simulink model "Noncoherent_BFSK"  (R2013a)
settings: Solver=ode45  StartTime=0.0  StopTime=32/(1200)  RelTol=1e-3
libraries: commrandsrc2 x1
settings Model: Creator=Cedric  LastModifiedBy=Cedric

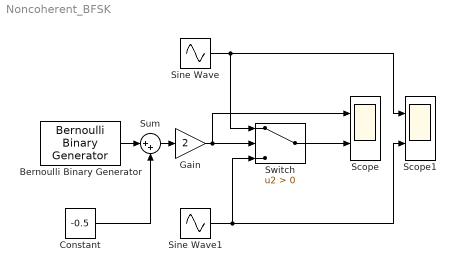
== system Noncoherent_BFSK ==
  Bernoulli Binary Generator : commrandsrc2/Bernoulli Binary Generator  P=0.5  seed=randseed  Ts=1/(1200)  frameBased=off  sampPerFrame=1  orient=off  outDataType=double
  Constant : Constant  Value=-0.5
  Gain : Gain  Gain=2
  Scope : Scope  NumInputPorts=2
      settings: YMin=-5~-5  YMax=5~5
  Scope1 : Scope  NumInputPorts=2
      settings: YMin=-5~-5  YMax=5~5
  Sine Wave : Sin  SineType=Sample based  Amplitude=5  Frequency=2*pi*1200  Samples=64  SampleTime=1/(1200*64)
  Sine Wave1 : Sin  SineType=Sample based  Amplitude=5  Frequency=2*pi*2200  Samples=64  SampleTime=1/(2200*64)
  Sum : Sum  Inputs=|++
  Switch : Switch  Criteria=u2 > Threshold
  wires:
  Sine Wave/1 -> Scope1/1, Switch/1
  Sine Wave1/1 -> Scope1/2, Switch/3
  Switch/1 -> Scope/2
  Constant/1 -> Sum/2
  Bernoulli Binary Generator/1 -> Sum/1
  Sum/1 -> Gain/1
  Gain/1 -> Scope/1, Switch/2
